simulink subsystem "LEDs"  (R2025b)
settings: Solver=VariableStepAuto  StartTime=0.0  StopTime=10.0  RelTol=1e-3
settings Model: Creator=JesseJabezArendse  LastModifiedBy=JesseJabezArendse
settings RTWCC: GPUComputeCapability=3.5

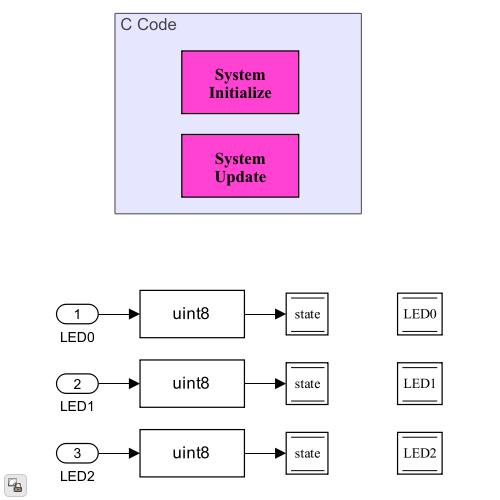
[thumbnail: Simulink's stored preview of the top-level diagram]
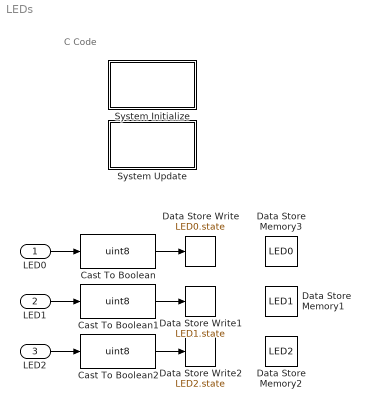
== system LEDs ==
  note: C Code
  LED0 : Inport
  LED1 : Inport  Port=2
  LED2 : Inport  Port=3
  Cast To Boolean : DataTypeConversion  OutDataTypeStr=uint8  SaturateOnIntegerOverflow=off  RndMeth=Floor
  Cast To Boolean1 : DataTypeConversion  OutDataTypeStr=uint8  SaturateOnIntegerOverflow=off  RndMeth=Floor
  Cast To Boolean2 : DataTypeConversion  OutDataTypeStr=uint8  SaturateOnIntegerOverflow=off  RndMeth=Floor
  Data Store Memory1 : DataStoreMemory  DataStoreName=LED1  WriteAfterWriteMsg=warning  ShowAdditionalParam=off  OutDataTypeStr=Bus: LED_t
  Data Store Memory2 : DataStoreMemory  DataStoreName=LED2  WriteAfterWriteMsg=warning  ShowAdditionalParam=off  OutDataTypeStr=Bus: LED_t
  Data Store Memory3 : DataStoreMemory  DataStoreName=LED0  WriteAfterWriteMsg=warning  ShowAdditionalParam=off  OutDataTypeStr=Bus: LED_t
  Data Store Write : DataStoreWrite  DataStoreName=LED0  DataStoreElements=LED0.state  IndexOptions=Index vector (dialog)  Indices=1  OutputSizes=1
  Data Store Write1 : DataStoreWrite  DataStoreName=LED1  DataStoreElements=LED1.state  IndexOptions=Index vector (dialog)  Indices=1  OutputSizes=1
  Data Store Write2 : DataStoreWrite  DataStoreName=LED2  DataStoreElements=LED2.state  IndexOptions=Index vector (dialog)  Indices=1  OutputSizes=1
  System Initialize : Subsystem  mask(System Initialize){ShowInLibBrowser=0}
      mask prompts: ShowInLibBrowser "Simulink:masks:CustCodeMaskParam1_MP"
      settings: CopyFcn=cccopyfcn(gcb)  OpenFcn=ccopenfcn('System Initialize Function')
      mask Help: eval('feval(''rtwprivate'',''rtwhelpview'',''rtw_sys_initialize_block'')');
      mask Display: disp('System\nInitialize');
  System Update : Subsystem  mask(System Update){ShowInLibBrowser=0}
      mask prompts: ShowInLibBrowser "Simulink:masks:CustCodeMaskParam1_MP"
      settings: CopyFcn=cccopyfcn(gcb)  OpenFcn=ccopenfcn('System Update Function')
      mask Help: eval('feval(''rtwprivate'',''rtwhelpview'',''rtw_sys_update_block'')');
      mask Display: disp('System\nUpdate');
  wires:
  LED0/1 -> Cast To Boolean/1
  LED1/1 -> Cast To Boolean1/1
  LED2/1 -> Cast To Boolean2/1
  Cast To Boolean/1 -> Data Store Write/1
  Cast To Boolean1/1 -> Data Store Write1/1
  Cast To Boolean2/1 -> Data Store Write2/1

== system LEDs/System Initialize ==

== system LEDs/System Update ==
